simulink model "rocket attempt"  (R2026a)
settings: Solver=VariableStepAuto
settings Model: Creator=tdxt  LastModifiedBy=tdxt

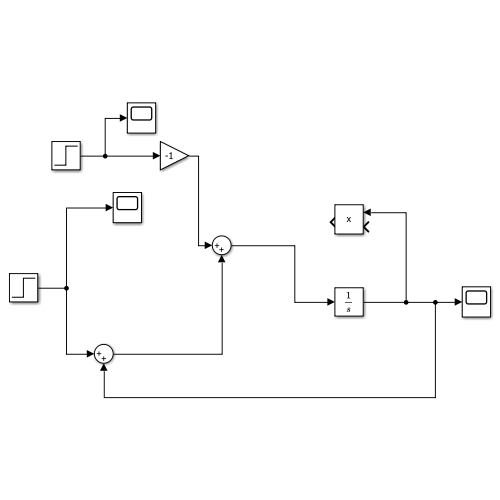
[thumbnail: Simulink's stored preview of the top-level diagram]
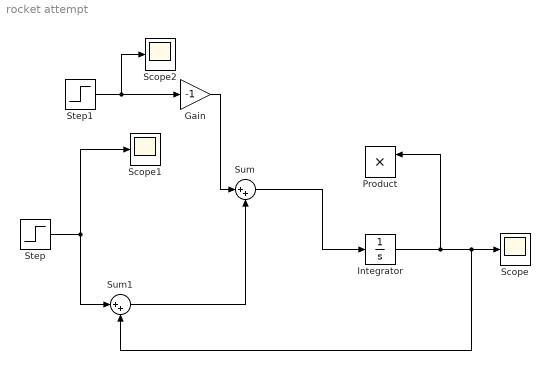
== system rocket attempt ==
  Gain : Gain  Gain=-1
  Integrator : Integrator
  Product : Product
  Scope : Scope
  Scope1 : Scope
      settings: ActiveDisplayYMinimum=-0.12499999999999997  ActiveDisplayYMaximum=1.125
  Scope2 : Scope
      settings: ActiveDisplayYMinimum=-0.12499999999999997  ActiveDisplayYMaximum=1.125  DataLoggingVariableName=ScopeData2
  Step : Step  SampleTime=0
  Step1 : Step  Time=6  SampleTime=0
  Sum : Sum  Inputs=|++
  Sum1 : Sum  Inputs=|++
  wires:
  Sum/1 -> Integrator/1
  Integrator/1 -> Product/1, Sum1/2, Scope/1
  Step/1 -> Sum1/1, Scope1/1
  Step1/1 -> Gain/1, Scope2/1
  Gain/1 -> Sum/1
  Sum1/1 -> Sum/2
